simulink model "Q1p9"  (R2018b)
settings: Solver=VariableStepAuto  StartTime=0.0  StopTime=0.5  RelTol=1e-3
values from neighbouring files (symbols this model uses):
  A = [0 1 0 0 0 0 ;  0 0 -10 0 -10 0; 0 0 0 1 0 0 ; 0 0 20 0 10 0 ; 0 0 0 0 0 1; 0 0 20 0 40 0]    [Q1part6.m]    (also in Q1part7.m; Q1part8.m; Q1part9.m)
  B = [0 1 0 -1 0 -2]'    [Q1part6.m]    (also in Q1part7.m; Q1part8.m; Q1part9.m)
  C = [0 0 1 0 0 0]    [Q1part6.m]    (also in Q1part7.m; Q1part8.m = [1 0 0 0 0 0; 0 0 1 0 0 0 ;0 0 0 0 1 0]; Q1part9.m = [1 0 0 0 0 0; 0 0 1 0 0 0 ;0 0 0 0 1 0])
  D = 0    [Q1part6.m]    (also in Q1part7.m; Q1part8.m = [-30 0 0 ; 0 -30 0 ;0 0 -30]; Q1part9.m = [-30 0 0 ; 0 -30 0 ;0 0 -30])
  f1 = [ 1     0     0 ... (first row only)    [Q1part8.m]    (also in Q1part9.m)
  f2 = [ 0     0     0 ... (first row only)    [Q1part8.m]    (also in Q1part9.m)
  k = k3    [Q1part6.m]    (also in Q1part7.m = qi*alphaA; Q1part9.m = qi*alphaA)
  R = L*B    [Q1part8.m]    (also in Q1part9.m = L2*B)
  T = phic*inv(phicC)    [Q1part6.m]    (also in Q1part8.m = A12+Lbar*A22-D*Lbar; Q1part9.m = A12+L*A22-D*L)
settings Model: Creator=Asus  LastModifiedBy=Asus

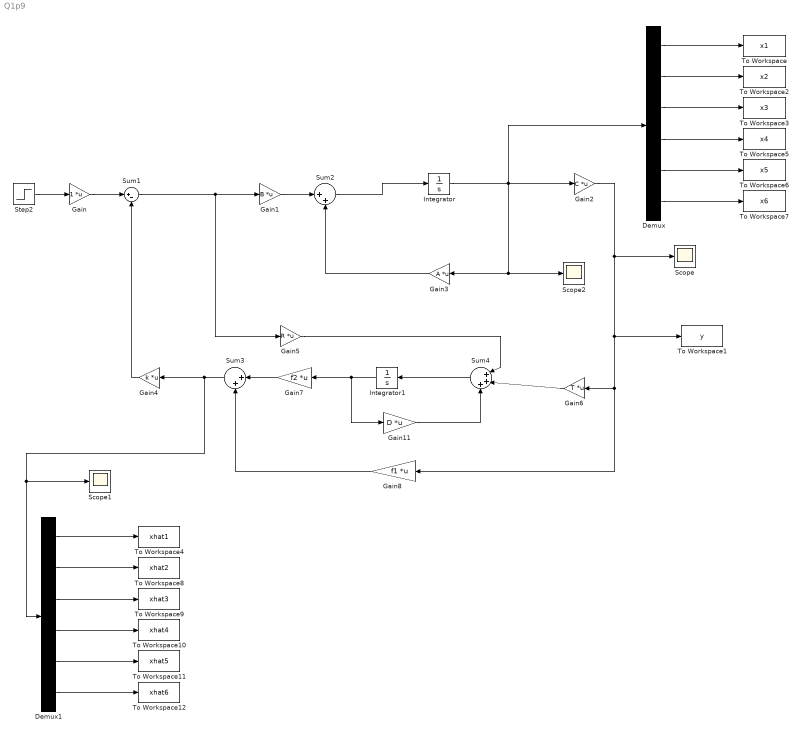
== system Q1p9 ==
  Demux : Demux  Outputs=6
  Demux1 : Demux  Outputs=6
  Gain : Gain  Multiplication=Matrix(K*u)
  Gain1 : Gain  Gain=B  Multiplication=Matrix(K*u)
  Gain11 : Gain  Gain=D  Multiplication=Matrix(K*u)
  Gain2 : Gain  Gain=C  Multiplication=Matrix(K*u)
  Gain3 : Gain  Gain=A  Multiplication=Matrix(K*u)
  Gain4 : Gain  Gain=k  Multiplication=Matrix(K*u)
  Gain5 : Gain  Gain=R  Multiplication=Matrix(K*u)
  Gain6 : Gain  Gain=T  Multiplication=Matrix(K*u)
  Gain7 : Gain  Gain=f2  Multiplication=Matrix(K*u)
  Gain8 : Gain  Gain=f1  Multiplication=Matrix(K*u)
  Integrator : Integrator  InitialCondition=[0 0 0.1 0 -0.1 0]
  Integrator1 : Integrator  InitialCondition=[0 0.5 -0.5]
  Scope : Scope
  Scope1 : Scope
  Scope2 : Scope
  Step2 : Step  Time=0  After=0  SampleTime=0
  Sum1 : Sum  Inputs=|+-
  Sum2 : Sum  Inputs=|++
  Sum3 : Sum  Inputs=|++
  Sum4 : Sum  Inputs=|+++
  To Workspace : ToWorkspace  VariableName=x1  SaveFormat=Timeseries  SampleTime=-1
  To Workspace1 : ToWorkspace  VariableName=y  SaveFormat=Timeseries  SampleTime=-1
  To Workspace10 : ToWorkspace  VariableName=xhat4  SaveFormat=Timeseries  SampleTime=-1
  To Workspace11 : ToWorkspace  VariableName=xhat5  SaveFormat=Timeseries  SampleTime=-1
  To Workspace12 : ToWorkspace  VariableName=xhat6  SaveFormat=Timeseries  SampleTime=-1
  To Workspace2 : ToWorkspace  VariableName=x2  SaveFormat=Timeseries  SampleTime=-1
  To Workspace3 : ToWorkspace  VariableName=x3  SaveFormat=Timeseries  SampleTime=-1
  To Workspace4 : ToWorkspace  VariableName=xhat1  SaveFormat=Timeseries  SampleTime=-1
  To Workspace5 : ToWorkspace  VariableName=x4  SaveFormat=Timeseries  SampleTime=-1
  To Workspace6 : ToWorkspace  VariableName=x5  SaveFormat=Timeseries  SampleTime=-1
  To Workspace7 : ToWorkspace  VariableName=x6  SaveFormat=Timeseries  SampleTime=-1
  To Workspace8 : ToWorkspace  VariableName=xhat2  SaveFormat=Timeseries  SampleTime=-1
  To Workspace9 : ToWorkspace  VariableName=xhat3  SaveFormat=Timeseries  SampleTime=-1
  wires:
  Gain5/1 -> Sum4/1
  Sum4/1 -> Integrator1/1
  Gain4/1 -> Sum1/2
  Gain8/1 -> Sum3/2
  Demux/4 -> To Workspace5/1
  Gain2/1 -> Gain6/1, Gain8/1, To Workspace1/1, Scope/1
  Integrator/1 -> Demux/1, Scope2/1, Gain3/1, Gain2/1
  Gain11/1 -> Sum4/3
  Gain6/1 -> Sum4/2
  Demux/1 -> To Workspace/1
  Integrator1/1 -> Gain11/1, Gain7/1
  Gain1/1 -> Sum2/1
  Gain/1 -> Sum1/1
  Gain7/1 -> Sum3/1
  Sum1/1 -> Gain1/1, Gain5/1
  Demux/5 -> To Workspace6/1
  Gain3/1 -> Sum2/2
  Demux/6 -> To Workspace7/1
  Demux/2 -> To Workspace2/1
  Sum2/1 -> Integrator/1
  Step2/1 -> Gain/1
  Demux/3 -> To Workspace3/1
  Demux1/2 -> To Workspace8/1
  Demux1/4 -> To Workspace10/1
  Demux1/6 -> To Workspace12/1
  Demux1/5 -> To Workspace11/1
  Demux1/3 -> To Workspace9/1
  Demux1/1 -> To Workspace4/1
  Sum3/1 -> Scope1/1, Demux1/1, Gain4/1
